simulink model "simulink_test"  (R2021b)
settings: Solver=VariableStepAuto  StartTime=0.0  StopTime=10.0  RelTol=1e-3
model workspace (MAT data in the model file):
  wn = 2
undefined symbols (not defined in the file or in its folder): zeta
settings Model: Creator=Studenci  LastModifiedBy=Studenci

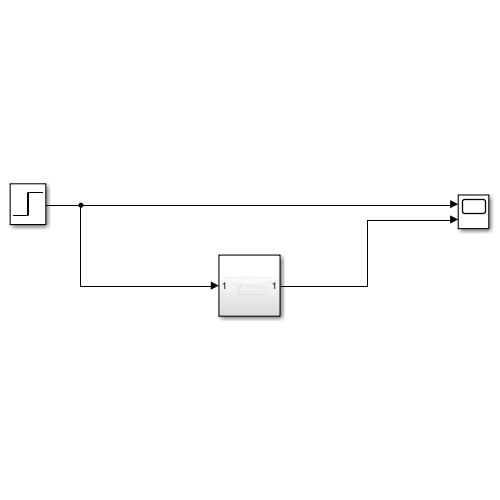
[thumbnail: Simulink's stored preview of the top-level diagram]
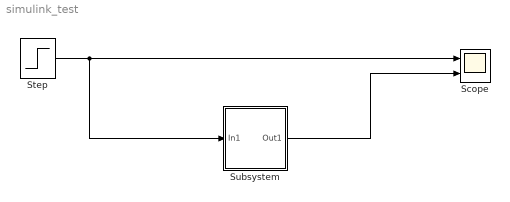
== system simulink_test ==
  Scope : Scope  NumInputPorts=2
  Step : Step  SampleTime=0
  Subsystem : Subsystem
  wires:
  Step/1 -> Subsystem/1(In1), Scope/1
  Subsystem/1(Out1) -> Scope/2

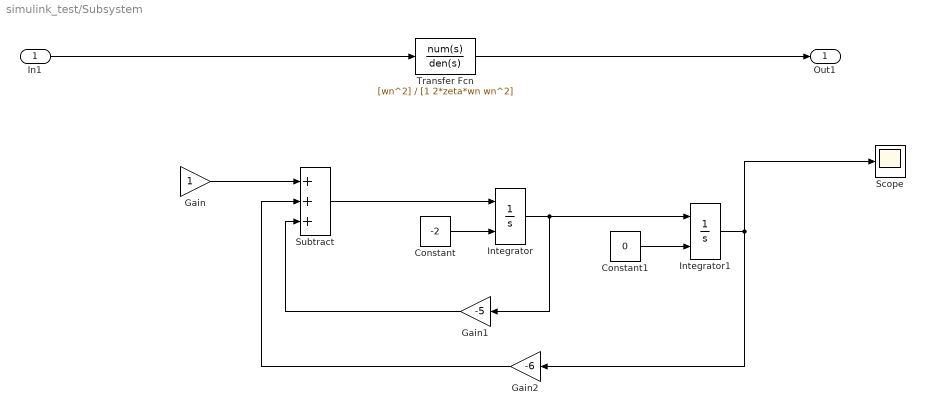
== system simulink_test/Subsystem ==
  In1 : Inport
  Constant : Constant  Value=-2
  Constant1 : Constant  Value=0
  Gain : Gain
  Gain1 : Gain  Gain=-5
  Gain2 : Gain  Gain=-6
  Integrator : Integrator  InitialConditionSource=external
  Integrator1 : Integrator  InitialConditionSource=external
  Scope : Scope
  Subtract : Sum  Inputs=+++
  Transfer Fcn : TransferFcn  Numerator=[wn^2]  Denominator=[1 2*zeta*wn wn^2]
  Out1 : Outport
  wires:
  In1/1 -> Transfer Fcn/1
  Transfer Fcn/1 -> Out1/1
  ? -> Gain/1
  Gain/1 -> Subtract/1
  Integrator/1 -> Integrator1/1, Gain1/1
  Constant/1 -> Integrator/2
  Gain1/1 -> Subtract/3
  Subtract/1 -> Integrator/1
  Integrator1/1 -> Gain2/1, Scope/1
  Constant1/1 -> Integrator1/2
  Gain2/1 -> Subtract/2
